simulink model "DomesticSolarTracker_LogicFlow"  (R2024b)
settings: Solver=VariableStepAuto  StartTime=0.0  StopTime=120  RelTol=1e-3
PreLoadFcn:
  | addpath(fullfile('WormAndGearConstraintSupport','Data'));
  | addpath(fullfile('WormAndGearConstraintSupport','Scripts'));
model workspace: external: MATLAB File WormAndGearConstraintParameters.m (data not in the file)
undefined symbols (not defined in the file): latitude, longitude, panelAzimuth, panelElevation, slewdrive, SPN1_MinGlobal, timeVector, X, Y, Z
libraries: sm_lib x27, nesl_utility x10, WormAndGearConstraintLibrary x8, fl_lib x6, spsSeriesRLCBranchLib x4, spsPVArrayLib x2, sps_lib x1, ee_lib x1, slpidlib x1
(part 2 of 2)

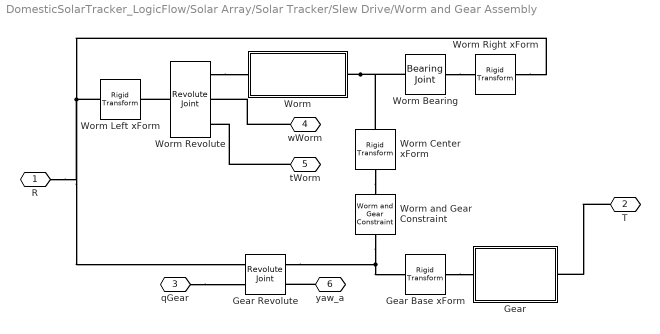
== system DomesticSolarTracker_LogicFlow/Solar Array/Solar Tracker/Slew Drive/Worm and Gear Assembly ==
  Gear : Subsystem  AncestorBlock=WormAndGearConstraintLibrary/Sliced Hollow Cylinder  mask(Sliced Hollow Cylinder){outerRadius=gearOuterRadius, thickness=gearThickness, length=gearLength, sliceThickness=gearSliceThickness, rho=gearRho, mainColor=gearColor, sliceColor=gearSliceColor}
      mask prompts: outerRadius "Outer Radius (m)"; thickness "Thickness (m)"; length "Length (m)"; sliceThickness "Slice Thickness (m)"; rho "Density (kg/m^3)"; mainColor "Main Color [r g b]"; sliceColor "Slice Color [r g b]"
      mask help:
      | This block models a hollow cylinder where a slice of the cylinder can be set to a different color.
      |
      | Port L corresponds to the left-hand end of the cylinder. Port R corresponds to the right-hand end of the cylinder.
      mask init:
      | points = 30;
      | 
      | innerRadius = outerRadius - thickness;
      | 
      | outerTheta = acos(0.5*sliceThickness / outerRadius);
      | 
      | rightOuterThetaVect = linspace(  -outerTheta,      outerTheta, points);
      | leftOuterThetaVect  = linspace(pi-outerTheta,   pi+outerTheta, points);
      | topOuterThetaVect   = linspace(   outerTheta,   pi-outerTheta, points);
      | botOuterThetaVect   = linspace(pi+outerTheta, 2*pi-outerTheta, points);
      | 
      | if (sliceThickness > 2*innerRadius)
      |   % The slice is wider than the hole
      |   rightCrossSection = [outerRadius*cos(rightOuterThetaVect);...
      |                        outerRadius*sin(rightOuterThetaVect)]';
      |   leftCrossSection  = [outerRadius*cos(leftOuterThetaVect);...
      |                        outerRadius*sin(leftOuterThetaVect)]';
      | 
      |   topInnerThetaVect = linspace(pi, 0, points);
      |   botInnerThetaVect = linspace(0, -pi, points);
      |   
      |   topCrossSection = [...
      |     outerRadius*cos(topOuterThetaVect) -0.5*sliceThickness innerRadius*cos(topInnerThetaVect) 0.5*sliceThickness;...
      |     outerRadius*sin(topOuterThetaVect) 0 innerRadius*sin(topInnerThetaVect) 0]';
      |   
      |   botCrossSection = [...
      |     outerRadius*cos(botOuterThetaVect) 0.5*sliceThickness innerRadius*cos(botInnerThetaVect) -0.5*sliceThickness;...
      |     outerRadius*sin(botOuterThetaVect) 0 innerRadius*sin(botInnerThetaVect) 0]';
      | else
      |   % The slicer is narrower than the hole
      |   innerTheta = acos(0.5*sliceThickness / innerRadius);
      |   
      |   rightInnerThetaVect = linspace(   innerTheta,    -innerTheta, points);
      |   leftInnerThetaVect  = linspace(pi+innerTheta,  pi-innerTheta, points);
      |   topInnerThetaVect   = linspace(pi-innerTheta,     innerTheta, points);
      |   botInnerThetaVect   = linspace(  -innerTheta, -pi+innerTheta, points);
      |   
      |   rightCrossSection = [...
      |     outerRadius*cos(rightOuterThetaVect) innerRadius*cos(rightInnerThetaVect);...
      |     outerRadius*sin(rightOuterThetaVect) innerRadius*sin(rightInnerThetaVect)]';
      |   leftCrossSection  = [...
      |     outerRadius*cos(leftOuterThetaVect)  innerRadius*cos(leftInnerThetaVect);...
      |     outerRadius*sin(leftOuterThetaVect)  innerRadius*sin(leftInnerThetaVect)]';
      |   topCrossSection   = [...
      |     outerRadius*cos(topOuterThetaVect)   innerRadius*cos(topInnerThetaVect);...
      |     outerRadius*sin(topOuterThetaVect)   innerRadius*sin(topInnerThetaVect)]';
      |   botCrossSection   = [...
      |     outerRadius*cos(botOuterThetaVect)   innerRadius*cos(botInnerThetaVect);...
      |     outerRadius*sin(botOuterThetaVect)   innerRadius*sin(botInnerThetaVect)]';
      | end
      mask DialogControl Tab1 Prompt: Dimensions
      mask DialogControl Tab2 Prompt: Material Properties
      mask Display:
      | image(fullfile('WormAndGearConstraintSupport','Images','HollowCylinder.png'));
      | port_label('lconn',1,'L');
      | port_label('rconn',1,'R');
  Gear Base xForm : sm_lib/Frames and Transforms/Rigid Transform  RotationMethod=None  FollAlignAxisA=+X  BaseAlignAxisA=+Y  FollAlignAxisB=+Y  BaseAlignAxisB=+Z  RotationStandardAxis=+Z  RotationAngle=0.0  RotationAngleUnits=deg  RotationArbitraryAxis=[0 0 1]  RotationSequenceAxes=FollowerAxes  RotationSequence=XYX  RotationSequenceAngles=[0 0 0]  RotationSequenceAnglesUnits=deg  RotationMatrix=[1 0 0; 0 1 0; 0 0 1]  Quaternion=[1 0 0 0]  TranslationMethod=StandardAxis  TranslationCartesianOffset=[0 0 0]  TranslationCartesianOffsetUnits=m  TranslationStandardAxis=-Z  TranslationStandardOffset=0.5*gearLength  TranslationStandardOffsetUnits=m  TranslationROffset=0  TranslationROffsetUnits=m  TranslationThetaOffset=0  TranslationThetaOffsetUnits=deg  TranslationZOffset=0  TranslationZOffsetUnits=m
  Gear Revolute : sm_lib/Joints/Revolute Joint  JointMode=Normal  CompositeWrenchDir=FollowerOnBase  CompositeWrenchFrame=BaseFrame  SenseConstraintForce=off  SenseConstraintTorque=off  SenseTotalForce=off  SenseTotalTorque=off  PositionTargetSpecify=off  PositionTargetPriority=High  PositionTargetValue=0  PositionTargetValueUnits=deg  VelocityTargetSpecify=off  VelocityTargetPriority=High  VelocityTargetValue=0  VelocityTargetValueUnits=deg/s  EquilibriumPosition=0  EquilibriumPositionUnits=deg  SpringStiffness=0  SpringStiffnessUnits=N*m/deg  DampingCoefficient=0  DampingCoefficientUnits=N*m/(deg/s)  LowerLimitSpecify=off  LowerLimitBound=-90  LowerLimitBoundUnits=deg  LowerLimitStiffness=1e4  LowerLimitStiffnessUnits=N*m/deg  LowerLimitDamping=10  LowerLimitDampingUnits=N*m/(deg/s)  LowerLimitTransitionRegionWidth=0.1  LowerLimitTransitionRegionWidthUnits=deg  UpperLimitSpecify=off  UpperLimitBound=90  UpperLimitBoundUnits=deg  UpperLimitStiffness=1e4  UpperLimitStiffnessUnits=N*m/deg  UpperLimitDamping=10  UpperLimitDampingUnits=N*m/(deg/s)  UpperLimitTransitionRegionWidth=0.1  UpperLimitTransitionRegionWidthUnits=deg  TorqueActuationMode=NoTorque  MotionActuationMode=InputMotion  SensePosition=on  SenseVelocity=off  SenseAcceleration=off  SenseTorqueForce=off  SenseLowerLimitTorqueForce=off  SenseUpperLimitTorqueForce=off
  Worm : Subsystem
      mask Display:
      | image(fullfile('WormAndGearConstraintSupport','Images','SlewDriveWorm.png'));
      | port_label('lconn',1,'S');
      | port_label('rconn',1,'B');
  Worm Bearing : sm_lib/Joints/Bearing Joint  JointMode=Normal  CompositeWrenchDir=FollowerOnBase  CompositeWrenchFrame=BaseFrame  SenseConstraintForce=off  SenseConstraintTorque=off  SenseTotalForce=off  SenseTotalTorque=off  PzPositionTargetSpecify=off  PzPositionTargetPriority=High  PzPositionTargetValue=0  PzPositionTargetValueUnits=m  PzVelocityTargetSpecify=off  PzVelocityTargetPriority=High  PzVelocityTargetValue=0  PzVelocityTargetValueUnits=m/s  PzEquilibriumPosition=0  PzEquilibriumPositionUnits=m  PzSpringStiffness=0  PzSpringStiffnessUnits=N/m  PzDampingCoefficient=0  PzDampingCoefficientUnits=N/(m/s)  PzLowerLimitSpecify=off  PzLowerLimitBound=-1  PzLowerLimitBoundUnits=m  PzLowerLimitStiffness=1e6  PzLowerLimitStiffnessUnits=N/m  PzLowerLimitDamping=1e3  PzLowerLimitDampingUnits=N/(m/s)  PzLowerLimitTransitionRegionWidth=1e-4  PzLowerLimitTransitionRegionWidthUnits=m  PzUpperLimitSpecify=off  PzUpperLimitBound=1  PzUpperLimitBoundUnits=m  PzUpperLimitStiffness=1e6  PzUpperLimitStiffnessUnits=N/m  PzUpperLimitDamping=1e3  PzUpperLimitDampingUnits=N/(m/s)  PzUpperLimitTransitionRegionWidth=1e-4  PzUpperLimitTransitionRegionWidthUnits=m  PzTorqueActuationMode=NoTorque  PzMotionActuationMode=ComputedMotion  PzSensePosition=off  PzSenseVelocity=off  PzSenseAcceleration=off  PzSenseTorqueForce=off  PzSenseLowerLimitTorqueForce=off  PzSenseUpperLimitTorqueForce=off  RxPositionTargetSpecify=off  RxPositionTargetPriority=High  RxPositionTargetValue=0  RxPositionTargetValueUnits=deg  RxVelocityTargetSpecify=off  RxVelocityTargetPriority=High  RxVelocityTargetValue=0  RxVelocityTargetValueUnits=deg/s  RxEquilibriumPosition=0  RxEquilibriumPositionUnits=deg  RxSpringStiffness=0  RxSpringStiffnessUnits=N*m/deg  RxDampingCoefficient=0  RxDampingCoefficientUnits=N*m/(deg/s)  RxLowerLimitSpecify=off  RxLowerLimitBound=-90  RxLowerLimitBoundUnits=deg  RxLowerLimitStiffness=1e4  RxLowerLimitStiffnessUnits=N*m/deg  RxLowerLimitDamping=10  RxLowerLimitDampingUnits=N*m/(deg/s)  RxLowerLimitTransitionRegionWidth=0.1  RxLowerLimitTransitionRegionWidthUnits=deg  RxUpperLimitSpecify=off  RxUpperLimitBound=90  RxUpperLimitBoundUnits=deg  RxUpperLimitStiffness=1e4  RxUpperLimitStiffnessUnits=N*m/deg  RxUpperLimitDamping=10  RxUpperLimitDampingUnits=N*m/(deg/s)  RxUpperLimitTransitionRegionWidth=0.1  RxUpperLimitTransitionRegionWidthUnits=deg  RxTorqueActuationMode=NoTorque  RxMotionActuationMode=ComputedMotion  RxSensePosition=off  RxSenseVelocity=off  RxSenseAcceleration=off  RxSenseTorqueForce=off  RxSenseLowerLimitTorqueForce=off  RxSenseUpperLimitTorqueForce=off  RyPositionTargetSpecify=off  RyPositionTargetPriority=High  RyPositionTargetValue=0  RyPositionTargetValueUnits=deg  RyVelocityTargetSpecify=off  RyVelocityTargetPriority=High  RyVelocityTargetValue=0  RyVelocityTargetValueUnits=deg/s  RyEquilibriumPosition=0  RyEquilibriumPositionUnits=deg  RySpringStiffness=0  RySpringStiffnessUnits=N*m/deg  RyDampingCoefficient=0  RyDampingCoefficientUnits=N*m/(deg/s)  RyLowerLimitSpecify=off  RyLowerLimitBound=-90  RyLowerLimitBoundUnits=deg  RyLowerLimitStiffness=1e4  RyLowerLimitStiffnessUnits=N*m/deg  RyLowerLimitDamping=10  RyLowerLimitDampingUnits=N*m/(deg/s)  RyLowerLimitTransitionRegionWidth=0.1  RyLowerLimitTransitionRegionWidthUnits=deg  RyUpperLimitSpecify=off  RyUpperLimitBound=90  RyUpperLimitBoundUnits=deg  RyUpperLimitStiffness=1e4  RyUpperLimitStiffnessUnits=N*m/deg  RyUpperLimitDamping=10  RyUpperLimitDampingUnits=N*m/(deg/s)  RyUpperLimitTransitionRegionWidth=0.1  RyUpperLimitTransitionRegionWidthUnits=deg  RyTorqueActuationMode=NoTorque  RyMotionActuationMode=ComputedMotion  RySensePosition=off  RySenseVelocity=off  RySenseAcceleration=off  RySenseTorqueForce=off  RySenseLowerLimitTorqueForce=off  RySenseUpperLimitTorqueForce=off  RzPositionTargetSpecify=off  RzPositionTargetPriority=High  RzPositionTargetValue=0  RzPositionTargetValueUnits=deg  RzVelocityTargetSpecify=off  RzVelocityTargetPriority=High  RzVelocityTargetValue=0  RzVelocityTargetValueUnits=deg/s  RzEquilibriumPosition=0  RzEquilibriumPositionUnits=deg  RzSpringStiffness=0  RzSpringStiffnessUnits=N*m/deg  RzDampingCoefficient=0  RzDampingCoefficientUnits=N*m/(deg/s)  RzLowerLimitSpecify=off  RzLowerLimitBound=-90  RzLowerLimitBoundUnits=deg  RzLowerLimitStiffness=1e4  RzLowerLimitStiffnessUnits=N*m/deg  RzLowerLimitDamping=10  RzLowerLimitDampingUnits=N*m/(deg/s)  RzLowerLimitTransitionRegionWidth=0.1  RzLowerLimitTransitionRegionWidthUnits=deg  RzUpperLimitSpecify=off  RzUpperLimitBound=90  RzUpperLimitBoundUnits=deg  RzUpperLimitStiffness=1e4  RzUpperLimitStiffnessUnits=N*m/deg  RzUpperLimitDamping=10  RzUpperLimitDampingUnits=N*m/(deg/s)  RzUpperLimitTransitionRegionWidth=0.1  RzUpperLimitTransitionRegionWidthUnits=deg  RzTorqueActuationMode=NoTorque  RzMotionActuationMode=ComputedMotion  RzSensePosition=off  RzSenseVelocity=off  RzSenseAcceleration=off  RzSenseTorqueForce=off  RzSenseLowerLimitTorqueForce=off  RzSenseUpperLimitTorqueForce=off
  Worm Revolute : sm_lib/Joints/Revolute Joint  JointMode=Normal  CompositeWrenchDir=FollowerOnBase  CompositeWrenchFrame=BaseFrame  SenseConstraintForce=off  SenseConstraintTorque=off  SenseTotalForce=off  SenseTotalTorque=off  PositionTargetSpecify=off  PositionTargetPriority=High  PositionTargetValue=0  PositionTargetValueUnits=deg  VelocityTargetSpecify=off  VelocityTargetPriority=High  VelocityTargetValue=0  VelocityTargetValueUnits=deg/s  EquilibriumPosition=0  EquilibriumPositionUnits=deg  SpringStiffness=0  SpringStiffnessUnits=N*m/deg  DampingCoefficient=bWormRevolute  DampingCoefficientUnits=N*m/(deg/s)  LowerLimitSpecify=off  LowerLimitBound=-90  LowerLimitBoundUnits=deg  LowerLimitStiffness=1e4  LowerLimitStiffnessUnits=N*m/deg  LowerLimitDamping=10  LowerLimitDampingUnits=N*m/(deg/s)  LowerLimitTransitionRegionWidth=0.1  LowerLimitTransitionRegionWidthUnits=deg  UpperLimitSpecify=off  UpperLimitBound=90  UpperLimitBoundUnits=deg  UpperLimitStiffness=1e4  UpperLimitStiffnessUnits=N*m/deg  UpperLimitDamping=10  UpperLimitDampingUnits=N*m/(deg/s)  UpperLimitTransitionRegionWidth=0.1  UpperLimitTransitionRegionWidthUnits=deg  TorqueActuationMode=ComputedTorque  MotionActuationMode=ComputedMotion  SensePosition=off  SenseVelocity=on  SenseAcceleration=off  SenseTorqueForce=on  SenseLowerLimitTorqueForce=off  SenseUpperLimitTorqueForce=off
  Worm Center xForm : sm_lib/Frames and Transforms/Rigid Transform  RotationMethod=None  FollAlignAxisA=+X  BaseAlignAxisA=+Y  FollAlignAxisB=+Y  BaseAlignAxisB=+Z  RotationStandardAxis=+Z  RotationAngle=0.0  RotationAngleUnits=deg  RotationArbitraryAxis=[0 0 1]  RotationSequenceAxes=FollowerAxes  RotationSequence=XYX  RotationSequenceAngles=[0 0 0]  RotationSequenceAnglesUnits=deg  RotationMatrix=[1 0 0; 0 1 0; 0 0 1]  Quaternion=[1 0 0 0]  TranslationMethod=StandardAxis  TranslationCartesianOffset=[0 0 0]  TranslationCartesianOffsetUnits=m  TranslationStandardAxis=-Z  TranslationStandardOffset=0.5*wormLength  TranslationStandardOffsetUnits=m  TranslationROffset=0  TranslationROffsetUnits=m  TranslationThetaOffset=0  TranslationThetaOffsetUnits=deg  TranslationZOffset=0  TranslationZOffsetUnits=m
  Worm Left xForm : sm_lib/Frames and Transforms/Rigid Transform  RotationMethod=AlignedAxes  FollAlignAxisA=+Z  BaseAlignAxisA=+X  FollAlignAxisB=+Y  BaseAlignAxisB=+Y  RotationStandardAxis=+Z  RotationAngle=0.0  RotationAngleUnits=deg  RotationArbitraryAxis=[0 0 1]  RotationSequenceAxes=FollowerAxes  RotationSequence=XYX  RotationSequenceAngles=[0 0 0]  RotationSequenceAnglesUnits=deg  RotationMatrix=[1 0 0; 0 1 0; 0 0 1]  Quaternion=[1 0 0 0]  TranslationMethod=Cartesian  TranslationCartesianOffset=wormLeftOffset  TranslationCartesianOffsetUnits=m  TranslationStandardAxis=+Z  TranslationStandardOffset=0  TranslationStandardOffsetUnits=m  TranslationROffset=0  TranslationROffsetUnits=m  TranslationThetaOffset=0  TranslationThetaOffsetUnits=deg  TranslationZOffset=0  TranslationZOffsetUnits=m
  Worm Right xForm : sm_lib/Frames and Transforms/Rigid Transform  RotationMethod=AlignedAxes  FollAlignAxisA=+Z  BaseAlignAxisA=+X  FollAlignAxisB=+Y  BaseAlignAxisB=+Y  RotationStandardAxis=+Z  RotationAngle=0.0  RotationAngleUnits=deg  RotationArbitraryAxis=[0 0 1]  RotationSequenceAxes=FollowerAxes  RotationSequence=XYX  RotationSequenceAngles=[0 0 0]  RotationSequenceAnglesUnits=deg  RotationMatrix=[1 0 0; 0 1 0; 0 0 1]  Quaternion=[1 0 0 0]  TranslationMethod=Cartesian  TranslationCartesianOffset=wormRightOffset  TranslationCartesianOffsetUnits=m  TranslationStandardAxis=+Z  TranslationStandardOffset=0  TranslationStandardOffsetUnits=m  TranslationROffset=0  TranslationROffsetUnits=m  TranslationThetaOffset=0  TranslationThetaOffsetUnits=deg  TranslationZOffset=0  TranslationZOffsetUnits=m
  Worm and Gear Constraint : sm_lib/Gears and Couplings/Gears/Worm and Gear Constraint  WormDirection=RightHand  WormLeadAngle=wormLeadAngle  WormLeadAngleUnits=deg  SpecificationMethod=PitchCircleRadii  CenterDistance=20  CenterDistanceUnits=cm  Ratio=1  WormRadius=wormRadius  WormRadiusUnits=m  GearRadius=gearOuterRadius  GearRadiusUnits=m
  R : PMIOPort  Side=Left
  T : PMIOPort  Port=2  Side=Right
  qGear : PMIOPort  Port=3  Side=Left
  wWorm : PMIOPort  Port=4  Side=Right
  tWorm : PMIOPort  Port=5  Side=Right
  yaw_a : PMIOPort  Port=6  Side=Right
  connections:
  qGear/RConn1 -- Gear Revolute/LConn2
  Worm Center xForm/RConn1 -- Worm and Gear Constraint/LConn1
  Worm Revolute/RConn1 -- Worm/LConn1
  Worm/RConn1 -- Worm Center xForm/LConn1 -- Worm Bearing/RConn1
  Worm Bearing/LConn1 -- Worm Right xForm/RConn1
  Worm Right xForm/LConn1 -- R/RConn1 -- Gear Revolute/LConn1 -- Worm Left xForm/LConn1
  Gear Base xForm/RConn1 -- Gear/LConn1
  Worm Revolute/LConn1 -- Worm Left xForm/RConn1
  Worm and Gear Constraint/RConn1 -- Gear Base xForm/LConn1 -- Gear Revolute/RConn1
  T/RConn1 -- Gear/RConn1
  wWorm/RConn1 -- Worm Revolute/RConn2
  tWorm/RConn1 -- Worm Revolute/RConn3
  yaw_a/RConn1 -- Gear Revolute/RConn2

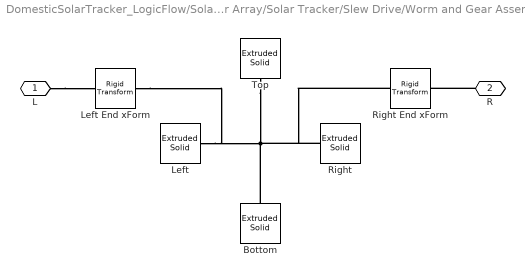
== system DomesticSolarTracker_LogicFlow/Solar Array/Solar Tracker/Slew Drive/Worm and Gear Assembly/Gear ==
  Bottom : sm_lib/Body Elements/Extruded Solid  ExtrusionType=General  PolygonNumSides=3  PolygonOuterRadius=1  PolygonOuterRadiusUnits=m  ExportEntireGeometry=off  ExtrusionCrossSection=botCrossSection  ExtrusionCrossSectionUnits=m  ExportConvexHullGeometry=off  ExtrusionLength=length  ExtrusionLengthUnits=m  InertiaType=CalculateFromGeometry  BasedOnType=Density  Density=rho  DensityUnits=kg/m^3  Mass=1  MassUnits=kg  CenterOfMass=[0 0 0]  CenterOfMassUnits=m  MomentsOfInertia=[1 1 1]  MomentsOfInertiaUnits=kg*m^2  ProductsOfInertia=[1 1 1]  ProductsOfInertiaUnits=kg*m^2  GraphicType=FromGeometry  MarkerShape=Sphere  MarkerSize=10  GraphicVisPropType=SimpleVisualProperties  GraphicDiffuseColor=sliceColor  GraphicOpacity=1.0  GraphicSpecularColor=[0.5 0.5 0.5 1.0]  GraphicAmbientColor=[0.15 0.15 0.15 1.0]  GraphicEmissiveColor=[0.0 0.0 0.0 1.0]  GraphicShininess=75  DoExposeReferenceFrame=on  SerializedFrames=<Frames/>
  Left : sm_lib/Body Elements/Extruded Solid  ExtrusionType=General  PolygonNumSides=3  PolygonOuterRadius=1  PolygonOuterRadiusUnits=m  ExportEntireGeometry=off  ExtrusionCrossSection=leftCrossSection  ExtrusionCrossSectionUnits=m  ExportConvexHullGeometry=off  ExtrusionLength=length  ExtrusionLengthUnits=m  InertiaType=CalculateFromGeometry  BasedOnType=Density  Density=rho  DensityUnits=kg/m^3  Mass=1  MassUnits=kg  CenterOfMass=[0 0 0]  CenterOfMassUnits=m  MomentsOfInertia=[1 1 1]  MomentsOfInertiaUnits=kg*m^2  ProductsOfInertia=[1 1 1]  ProductsOfInertiaUnits=kg*m^2  GraphicType=FromGeometry  MarkerShape=Sphere  MarkerSize=10  GraphicVisPropType=SimpleVisualProperties  GraphicDiffuseColor=mainColor  GraphicOpacity=1.0  GraphicSpecularColor=[0.5 0.5 0.5 1.0]  GraphicAmbientColor=[0.15 0.15 0.15 1.0]  GraphicEmissiveColor=[0.0 0.0 0.0 1.0]  GraphicShininess=75  DoExposeReferenceFrame=on  SerializedFrames=<Frames/>
  Left End xForm : sm_lib/Frames and Transforms/Rigid Transform  RotationMethod=None  FollAlignAxisA=+X  BaseAlignAxisA=+Y  FollAlignAxisB=+Y  BaseAlignAxisB=+Z  RotationStandardAxis=+Z  RotationAngle=0.0  RotationAngleUnits=deg  RotationArbitraryAxis=[0 0 1]  RotationSequenceAxes=FollowerAxes  RotationSequence=XYX  RotationSequenceAngles=[0 0 0]  RotationSequenceAnglesUnits=deg  RotationMatrix=[1 0 0; 0 1 0; 0 0 1]  Quaternion=[1 0 0 0]  TranslationMethod=StandardAxis  TranslationCartesianOffset=[0 0 0]  TranslationCartesianOffsetUnits=m  TranslationStandardAxis=-Z  TranslationStandardOffset=0.5*length  TranslationStandardOffsetUnits=m  TranslationROffset=0  TranslationROffsetUnits=m  TranslationThetaOffset=0  TranslationThetaOffsetUnits=deg  TranslationZOffset=0  TranslationZOffsetUnits=m
  Right : sm_lib/Body Elements/Extruded Solid  ExtrusionType=General  PolygonNumSides=3  PolygonOuterRadius=1  PolygonOuterRadiusUnits=m  ExportEntireGeometry=off  ExtrusionCrossSection=rightCrossSection  ExtrusionCrossSectionUnits=m  ExportConvexHullGeometry=off  ExtrusionLength=length  ExtrusionLengthUnits=m  InertiaType=CalculateFromGeometry  BasedOnType=Density  Density=rho  DensityUnits=kg/m^3  Mass=1  MassUnits=kg  CenterOfMass=[0 0 0]  CenterOfMassUnits=m  MomentsOfInertia=[1 1 1]  MomentsOfInertiaUnits=kg*m^2  ProductsOfInertia=[1 1 1]  ProductsOfInertiaUnits=kg*m^2  GraphicType=FromGeometry  MarkerShape=Sphere  MarkerSize=10  GraphicVisPropType=SimpleVisualProperties  GraphicDiffuseColor=mainColor  GraphicOpacity=1.0  GraphicSpecularColor=[0.5 0.5 0.5 1.0]  GraphicAmbientColor=[0.15 0.15 0.15 1.0]  GraphicEmissiveColor=[0.0 0.0 0.0 1.0]  GraphicShininess=75  DoExposeReferenceFrame=on  SerializedFrames=<Frames/>
  Right End xForm : sm_lib/Frames and Transforms/Rigid Transform  RotationMethod=None  FollAlignAxisA=+X  BaseAlignAxisA=+Y  FollAlignAxisB=+Y  BaseAlignAxisB=+Z  RotationStandardAxis=+Z  RotationAngle=0.0  RotationAngleUnits=deg  RotationArbitraryAxis=[0 0 1]  RotationSequenceAxes=FollowerAxes  RotationSequence=XYX  RotationSequenceAngles=[0 0 0]  RotationSequenceAnglesUnits=deg  RotationMatrix=[1 0 0; 0 1 0; 0 0 1]  Quaternion=[1 0 0 0]  TranslationMethod=StandardAxis  TranslationCartesianOffset=[0 0 0]  TranslationCartesianOffsetUnits=m  TranslationStandardAxis=+Z  TranslationStandardOffset=0.5*length  TranslationStandardOffsetUnits=m  TranslationROffset=0  TranslationROffsetUnits=m  TranslationThetaOffset=0  TranslationThetaOffsetUnits=deg  TranslationZOffset=0  TranslationZOffsetUnits=m
  Top : sm_lib/Body Elements/Extruded Solid  ExtrusionType=General  PolygonNumSides=3  PolygonOuterRadius=1  PolygonOuterRadiusUnits=m  ExportEntireGeometry=off  ExtrusionCrossSection=topCrossSection  ExtrusionCrossSectionUnits=m  ExportConvexHullGeometry=off  ExtrusionLength=length  ExtrusionLengthUnits=m  InertiaType=CalculateFromGeometry  BasedOnType=Density  Density=rho  DensityUnits=kg/m^3  Mass=1  MassUnits=kg  CenterOfMass=[0 0 0]  CenterOfMassUnits=m  MomentsOfInertia=[1 1 1]  MomentsOfInertiaUnits=kg*m^2  ProductsOfInertia=[1 1 1]  ProductsOfInertiaUnits=kg*m^2  GraphicType=FromGeometry  MarkerShape=Sphere  MarkerSize=10  GraphicVisPropType=SimpleVisualProperties  GraphicDiffuseColor=sliceColor  GraphicOpacity=1.0  GraphicSpecularColor=[0.5 0.5 0.5 1.0]  GraphicAmbientColor=[0.15 0.15 0.15 1.0]  GraphicEmissiveColor=[0.0 0.0 0.0 1.0]  GraphicShininess=75  DoExposeReferenceFrame=on  SerializedFrames=<Frames/>
  L : PMIOPort  Side=Left
  R : PMIOPort  Port=2  Side=Right
  connections:
  L/RConn1 -- Left End xForm/RConn1
  Top/RConn1 -- Bottom/RConn1 -- Right/RConn1 -- Right End xForm/LConn1 -- Left End xForm/LConn1 -- Left/RConn1
  R/RConn1 -- Right End xForm/RConn1

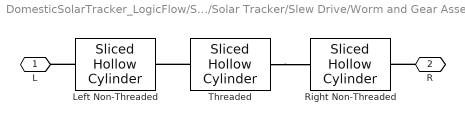
== system DomesticSolarTracker_LogicFlow/Solar Array/Solar Tracker/Slew Drive/Worm and Gear Assembly/Worm ==
  Left Non-Threaded : WormAndGearConstraintLibrary/Sliced Hollow Cylinder  outerRadius=wormNonThreadedRadius  thickness=wormNonThreadedThickness  length=wormNonThreadedLength  sliceThickness=wormSliceProportion*wormNonThreadedRadius  rho=wormRho  mainColor=wormColor  sliceColor=wormSliceColor
  Right Non-Threaded : WormAndGearConstraintLibrary/Sliced Hollow Cylinder  outerRadius=wormNonThreadedRadius  thickness=wormNonThreadedThickness  length=wormNonThreadedLength  sliceThickness=wormSliceProportion*wormNonThreadedRadius  rho=wormRho  mainColor=wormColor  sliceColor=wormSliceColor
  Threaded : WormAndGearConstraintLibrary/Sliced Hollow Cylinder  outerRadius=wormRadius  thickness=wormThreadedThickness  length=wormThreadedLength  sliceThickness=wormSliceProportion*wormRadius  rho=wormRho  mainColor=wormColor  sliceColor=wormSliceColor
  L : PMIOPort  Side=Left
  R : PMIOPort  Port=2  Side=Right
  connections:
  Threaded/LConn1 -- Left Non-Threaded/RConn1
  Threaded/RConn1 -- Right Non-Threaded/LConn1
  R/RConn1 -- Right Non-Threaded/RConn1
  Left Non-Threaded/LConn1 -- L/RConn1

== matlab function DomesticSolarTracker_LogicFlow/MATLAB Function1 ==
  data: timeVector input; solarTime output; irradianceEntry output; stopSim output
function [solarTime, irradianceEntry, stopSim] = dataSync(timeVector)
    % Sync solar position and solar irradiance with a counter 
    % using a persistent counter that increments every call.
    persistent counter 
    % Initialize counter on first call
    if isempty(counter)
        counter = 1;
    end
    % For solarTime we still output the current time-of-day (seconds)
    solarTime = timeVector(counter,:);

    % Convert the second-based counter into a minute-based index.
    % This index will be constant for 60 consecutive calls (seconds).
    irradianceEntry = floor((counter - 1) / 60) + 1;

    % Increment counter if there are more rows. Otherwise signal simulation stop.
    rows = size(timeVector, 1);
    if counter < rows
        counter = counter + 1;
        stopSim = false;
    else
        stopSim = true;
    end
end

== matlab function DomesticSolarTracker_LogicFlow/MATLAB Function ==
  data latitude settings: description=Year input
  data: latitude input double size=1; azimuth output size=1; longitude input double size=1; timeVector input double size=[1 6]; elevation output double size=1
function [azimuth, elevation] = calculateSolarPosition(latitude, longitude, timeVector)
    year = timeVector(1);
    month = timeVector(2);
    day = timeVector(3);
    hour = timeVector(4);
    minute = timeVector(5);
    second = timeVector(6);

    % Calculate Julian Date
    JD = calculateJulianDate(year, month, day, hour, minute, second);
    
    % Calculate days since J2000.0
    n = daysSinceJ2000(JD);
    
    % Calculate mean longitude of the sun
    L = meanLongitudeSun(n);
    
    % Calculate mean anomaly of the sun
    g = meanAnomalySun(n);
    
    % Calculate ecliptic longitude of the sun
    lambda = eclipticLongitudeSun(L, g);
    
    % Calculate obliquity of the ecliptic
    epsilon = obliquityEcliptic(n);
    
    % Calculate right ascension and declination of the sun
    [alpha, delta] = rightAscensionDeclination(lambda, epsilon);
    
    % Calculate local sidereal time
    LST = localSiderealTime(n, longitude, hour, minute, second);
    
    % Calculate hour angle
    H = hourAngle(LST, alpha);
    
    % Calculate elevation and azimuth angles (with azimuth referenced to north)
    [elevation, azimuth] = solarElevationAzimuth(latitude, delta, H);
end

% Helper functions
function JD = calculateJulianDate(year, month, day, hour, minute, second)
    if month <= 2
        year = year - 1;
        month = month + 12;
    end
    A = floor(year / 100);
    B = 2 - A + floor(A / 4);
    JD = floor(365.25 * (year + 4716)) + floor(30.6001 * (month + 1)) + day + B - 1524.5 ...
        + (hour + minute / 60 + second / 3600) / 24;
end

function n = daysSinceJ2000(JD)
    JD_J2000 = 2451545.0;  % Julian Date of J2000.0
    n = JD - JD_J2000;
end

function L = meanLongitudeSun(n)
    L = mod(280.460 + 0.9856474 * n, 360);
end

function g = meanAnomalySun(n)
    g = mod(357.528 + 0.9856003 * n, 360);
end

function lambda = eclipticLongitudeSun(L, g)
    lambda = mod(L + 1.915 * sind(g) + 0.020 * sind(2 * g), 360);
end

function epsilon = obliquityEcliptic(n)
    epsilon = 23.439 - 0.0000004 * n;
end

function [alpha, delta] = rightAscensionDeclination(lambda, epsilon)
    alpha = atan2d(cosd(epsilon) * sind(lambda), cosd(lambda));
    delta = asind(sind(epsilon) * sind(lambda));
end

function LST = localSiderealTime(n, longitude, hour, minute, second)
    GMST = mod(6.697374558 + 0.06570982441908 * n + (hour + minute / 60 + second / 3600) * 1.00273790935, 24);
    LST = mod(GMST * 15 + longitude, 360);
end

function H = hourAngle(LST, alpha)
    H = mod(LST - alpha, 360);
end


function [elevation, azimuth] = solarElevationAzimuth(latitude, delta, H)
    elevation = asind(sind(latitude) * sind(delta) + cosd(latitude) * cosd(delta) * cosd(H));
    azimuth = mod(atan2d(sind(H), cosd(H) * sind(latitude) - tand(delta) * cosd(latitude)) + 180, 360);
end

== matlab function DomesticSolarTracker_LogicFlow/PV Generation /MATLAB Function1 ==
  data: Irradiance input; EffectiveIrradiance output; SunAzimuth input; SunElevation input; PanelAzimuth input; PanelElevation input
 function EffectiveIrradiance = fcn(Irradiance,SunAzimuth,SunElevation,PanelAzimuth,PanelElevation)

% Convert spherical angles to cartesian coordinates
SunVector = [cosd(SunElevation)*sind(SunAzimuth), ...
             cosd(SunElevation)*cosd(SunAzimuth), ...
             sind(SunElevation)];
PanelNormal = [cosd(PanelElevation)*sind(PanelAzimuth), ...
               cosd(PanelElevation)*cosd(PanelAzimuth), ...
               sind(PanelElevation)];

% Get Cosine Angle of Incidence via Dot Product
Cos_Incidence = dot(SunVector,PanelNormal);

% Clamp Between 1 and 0 to Avoid Negitive Values
Cos_Incidence = max(Cos_Incidence,0);

% Scale Irradiance by Cosine Angle of Incidence 
EffectiveIrradiance = Irradiance * Cos_Incidence;
end

== stateflow chart DomesticSolarTracker_LogicFlow/Solar Array/stateflow logic chart ==
  state Cloudy
    entry:
    hold_yaw  = yaw ;
    during :
    yaw_upd = hold_yaw;
    exit:
    yaw_upd = hold_yaw;
  state Daytime
    during :
    yaw_upd = yaw;
  (default) -> Daytime
  Daytime -> Cloudy : [abs(yaw)>= 2.7 && irradiance < 450 ]
  Cloudy -> Daytime : [irradiance>= 450]
  data: yaw input; yaw_upd output; hold_yaw local double size=1; hold_pitch local double size=1; irradiance input

== matlab function DomesticSolarTracker_LogicFlow/PV Generation /MATLAB Function ==
  data: Irradiance input; EffectiveIrradiance output; SunAzimuth input; SunElevation input; PanelAzimuth input; PanelElevation input
function EffectiveIrradiance = fcn(Irradiance,SunAzimuth,SunElevation,PanelAzimuth,PanelElevation)

    SunAzimuth = mod(SunAzimuth + 180, 360);
    PanelAzimuth = mod(PanelAzimuth + 180, 360);

% Convert spherical angles to cartesian coordinates
SunVector = [cosd(SunElevation)*sind(SunAzimuth), ...
             cosd(SunElevation)*cosd(SunAzimuth), ...
             sind(SunElevation)];
PanelNormal = [cosd(PanelElevation)*sind(PanelAzimuth), ...
               cosd(PanelElevation)*cosd(PanelAzimuth), ...
               sind(PanelElevation)];

% Get Cosine Angle of Incidence via Dot Product
Cos_Incidence = dot(SunVector,PanelNormal);

% Clamp Between 1 and 0 to Avoid Negitive Values
Cos_Incidence = max(Cos_Incidence,0);

% Scale Irradiance by Cosine Angle of Incidence 
EffectiveIrradiance = Irradiance * Cos_Incidence;
end
